simulink model "drive_test"  (R2016a)
settings: Solver=FixedStepAuto  StartTime=0.0  StopTime=100  FixedStep=0.001  RelTol=1e-3
libraries: tinbot x1
settings Model: Creator=maximilian  LastModifiedBy=maximilian

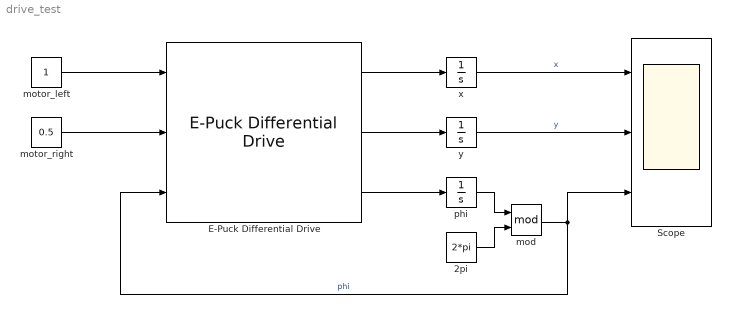
== system drive_test ==
  2pi : Constant  Value=2*pi
  E-Puck Differential Drive : tinbot/E-Puck Differential Drive  SystemSampleTime=-1
  Scope : Scope  NumInputPorts=3
  mod : Math  Operator=mod  SaturateOnIntegerOverflow=on
  motor_left : Constant
  motor_right : Constant  Value=0.5
  phi : Integrator
  x : Integrator
  y : Integrator
  wires:
  E-Puck Differential Drive/1 -> x/1
  motor_left/1 -> E-Puck Differential Drive/1
  motor_right/1 -> E-Puck Differential Drive/2
  x/1 -> Scope/1  "x"
  E-Puck Differential Drive/2 -> y/1
  E-Puck Differential Drive/3 -> phi/1
  y/1 -> Scope/2  "y"
  phi/1 -> mod/1
  mod/1 -> E-Puck Differential Drive/3, Scope/3  "phi"
  2pi/1 -> mod/2
